simulink model "linear_ss_control"  (R2019b)
settings: Solver=ode45  StartTime=0.0  StopTime=5700.0  MaxStep=0.01  RelTol=1e-8
settings Model: Creator=Hector  LastModifiedBy=Hector

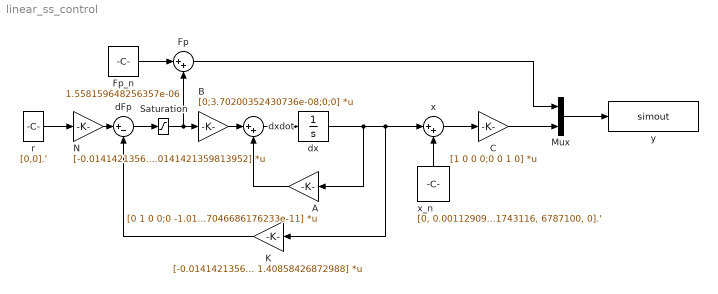
== system linear_ss_control ==
  A : Gain  Gain=[0 1 0 0;0 -1.01409337235247e-10 -1.70834505909243e-20 -3.36920663455173e-10;0 0 0 1;0 15365.0510962495 3.88260240702825e-06 -5.07046686176233e-11]  Multiplication=Matrix(K*u)
  B : Gain  Gain=[0;3.70200352430736e-08;0;0]  Multiplication=Matrix(K*u)
  C : Gain  Gain=[1 0 0 0;0 0 1 0]  Multiplication=Matrix(K*u)
  Fp : Sum  Inputs=|++
  Fp_n : Constant  Value=1.558159648256357e-06
  K : Gain  Gain=[-0.0141421356317003 1081321.55987828 0.0144153756634905 1.40858426872988]  Multiplication=Matrix(K*u)
  Mux : Mux  Inputs=2
  N : Gain  Gain=[-0.0141421356317003 0.0141421359813952]  Multiplication=Matrix(K*u)
  Saturation : Saturate  UpperLimit=21.558159648256357e-06  LowerLimit=-1.558159648256357e-06
  dFp : Sum  Inputs=|+-
  dx : Integrator  InitialCondition=[0, 0, -1*10^-3, 0].'
  dxdot : Sum  Inputs=|++
  r : Constant  Value=[0,0].'
  x : Sum  Inputs=|++
  x_n : Constant  Value=[0, 0.001129091743116, 6787100, 0].'
  y : ToWorkspace  VariableName=simout  SaveFormat=Timeseries  SampleTime=-1
  wires:
  dx/1 -> x/1, K/1, A/1
  dxdot/1 -> dx/1
  A/1 -> dxdot/2
  x/1 -> C/1
  x_n/1 -> x/2
  B/1 -> dxdot/1
  K/1 -> dFp/2
  Fp_n/1 -> Fp/1
  dFp/1 -> Saturation/1
  N/1 -> dFp/1
  Mux/1 -> y/1
  C/1 -> Mux/2
  Fp/1 -> Mux/1
  r/1 -> N/1
  Saturation/1 -> Fp/2, B/1
